simulink model "One_Phase_Uncontrolled_Bridge_Rectifier"  (R2017b)
settings: Solver=VariableStepAuto  StartTime=0.0  StopTime=1.0  MaxStep=1e-4  RelTol=1e-3
libraries: powerlib x16, powerlib_meascontrol x3
settings Model: Creator=DELL  LastModifiedBy=DELL

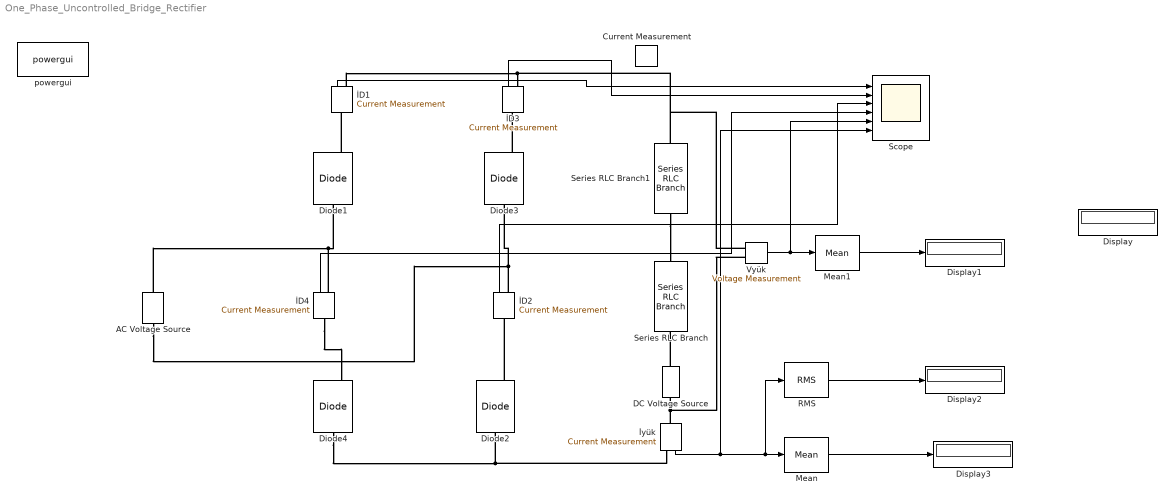
== system One_Phase_Uncontrolled_Bridge_Rectifier ==
  AC Voltage Source : powerlib/Electrical Sources/AC Voltage Source  Amplitude=220*(2^0.5)  Phase=0  Frequency=50  SampleTime=0  Measurements=None  BusType=swing  Pref=10e3  Qref=0  Qmin=-inf  Qmax=+inf
  Current Measurement : powerlib/Measurements/Current Measurement  PhasorSimulation=off  OutputType=Complex  PSBequivalent=0
  DC Voltage Source : powerlib/Electrical Sources/DC Voltage Source  Amplitude=100  Measurements=None
  Diode{1..4} (4 alike) : powerlib/Power Electronics/Diode  Ron=0.001  Lon=0  Vf=0.8  IC=0  UseSnubber=0  Rs=500  Cs=250e-9  Measurements=on
  Display{,1..3} (4 alike) : Display
  Mean : powerlib_meascontrol/Measurements/Mean  Freq=50  Vinit=0  Ts=0
  Mean1 : powerlib_meascontrol/Measurements/Mean  Freq=50  Vinit=0  Ts=0
  RMS : powerlib_meascontrol/Measurements/RMS  TrueRMS=on  Freq=50  RMSInit=120  Ts=0
  Scope : Scope  NumInputPorts=6
  Series RLC Branch : powerlib/Elements/Series RLC Branch  LConnTagsString=__new0  RConnTagsString=__new0  BranchType=L  Resistance=1  Inductance=10e-3  SetiL0=off  InitialCurrent=0  Capacitance=1e-6  Setx0=off  InitialVoltage=0  Measurements=None
  Series RLC Branch1 : powerlib/Elements/Series RLC Branch  LConnTagsString=__new0  RConnTagsString=__new0  BranchType=R  Resistance=10  Inductance=1e-3  SetiL0=off  InitialCurrent=0  Capacitance=1e-6  Setx0=off  InitialVoltage=0  Measurements=None
  Vyük : powerlib/Measurements/Voltage Measurement  PhasorSimulation=off  OutputType=Complex  PSBequivalent=0
  powergui : powerlib/powergui  Priority=1  SimulationMode=Continuous  SampleTime=50e-6  frequency=60  Iterations=50  frequencyindice=50  Pbase=100e6  ErrMax=1e-4  UnitsV=kV  UnitsW=MW  buscounter=0  FunctionMessages=off  echomessages=off  EnableUseOfTLC=off  CurrentSourceSwitches=off  DisableSnubberDevices=off  DisableRonSwitches=off  DisableVfSwitches=off  DisplayEquations=off  SolverType=Tustin/Backward Euler (TBE)  Interpol=off  ExternalGateDelay=off  methode=off  Ts=100  x0status=blocks  SPID=on  SwTol=0  HookPort=off  RestoreLinks=warning  ResistiveCurrentMeasurement=off  Frange=[0:2:500]  Ylog=off  Xlog=on  ShowGrid=off  save=off  variable=ZData  structure=0  ZoomFFT=off  StartTime=0.0  cycles=1  DisplayStyle=1  fundamental=60  FreqAxis=off  MaxFrequency=1000  frequencyindicesteady=1  RmsSteady=1  display=off
  İD{1..4} (4 alike) : powerlib/Measurements/Current Measurement  PhasorSimulation=off  OutputType=Complex  PSBequivalent=0
  İyük : powerlib/Measurements/Current Measurement  PhasorSimulation=off  OutputType=Complex  PSBequivalent=0
  wires:
  Mean1/1 -> Display1/1
  Vyük/1 -> Scope/5, Mean1/1
  İyük/1 -> Scope/6, RMS/1, Mean/1
  Mean/1 -> Display3/1
  RMS/1 -> Display2/1
  İD1/1 -> Scope/1
  İD3/1 -> Scope/2
  İD2/1 -> Scope/3
  İD4/1 -> Scope/4
  connections:
  İD4/LConn1 -- Diode4/RConn1
  AC Voltage Source/RConn1 -- Diode1/LConn1 -- İD4/RConn1
  Diode1/RConn1 -- İD1/LConn1
  İD1/RConn1 -- Vyük/LConn1 -- Series RLC Branch1/RConn1 -- İD3/RConn1
  Diode3/RConn1 -- İD3/LConn1
  Series RLC Branch1/LConn1 -- Series RLC Branch/RConn1
  DC Voltage Source/RConn1 -- Series RLC Branch/LConn1
  İyük/LConn1 -- Vyük/LConn2 -- DC Voltage Source/LConn1
  İyük/RConn1 -- Diode4/LConn1 -- Diode2/LConn1
  Diode2/RConn1 -- İD2/LConn1
  İD2/RConn1 -- AC Voltage Source/LConn1 -- Diode3/LConn1
